simulink model "IEEE34bus_v2019b_Discrete_ZIPload"  (R2019b)
settings: Solver=ode4  StartTime=0.0  StopTime=5  FixedStep=Ts  MaxStep=1e-4  RelTol=1e-4
InitFcn:
  | a=1; % Loading Factor
  | Ts=50e-6;
  | % phase to sequence conversion of RXB matrices
  | c=1*exp(sqrt(-1)*(120*pi/180));
  | T=[1 1 1;1 c*c c;1 c c*c];
  | Tinv=1/3*[1 1 1;1 c c*c;1 c*c c];
  | 
  | % Simulation data for the IEEE 34 Node Test Feeder model
  | mi2km = 1.60934;%  miles to km conversion
  | ft2km = 0.0003048; % feet to km conversion
  | ms2F = 1*1e-6/(2*pi*60);% microsiemens to Farads conversion
  | 
  | %% Configuration 300 - series reactance - ohm/mile
  | R_300 = [1.3368 0.2101 0.2130;0.2101 1.3238 0.2066;0.2130 0.2066 1.3294];
  | X_300 = [1.3343 0.5779 0.5015;0.5779 1.3569 0.4591;0.5015 0.4591 1.3471];
  | % charging susceptance - microsiemens/mile
  | B_300 = [5.3350 -1.5313 -0.9943;-1.5313 5.0979 -0.6212;-0.9943 -0.6212 4.8880];
  | 
  | R_300 = R_300/mi2km;
  | Rseq=Tinv*R_300*T;
  | R1_300=Rseq(2,2);R0_300=Rseq(1,1);
  | 
  | L_300 = (X_300/(2*pi*60))/mi2km;
  | Lseq=Tinv*L_300*T;
  | L1_300=Lseq(2,2);L0_300=Lseq(1,1);
  | 
  | C_300 =(B_300*ms2F)/mi2km;
  | Cseq=Tinv*C_300*T;
  | C1_300=Cseq(2,2);C0_300=Cseq(1,1);
  | 
  | %% Configuration 301 - series reactance - ohm/mile
  | R_301 = [1.9300 0.2327 0.2359;0.2327 1.9157 0.2288;0.2359 0.2288 1.9219];
  | X_301 = [1.4115 0.6442 0.5691;0.6442 1.4281 0.5238;0.5691 0.5238 1.4209];
  | % charging susceptance - microsiemens/mile
  | B_301 = [5.1207 -1.4364 -0.9402;-1.4364 4.9055 -0.5951;-0.9402 -0.5951 4.7154];
  | 
  | R_301 = R_301/mi2km;
  | Rseq=Tinv*R_301*T;
  | R1_301=Rseq(2,2);R0_301=Rseq(1,1);
  | 
  | L_301 = (X_301/(2*pi*60))/mi2km;
  | Lseq=Tinv*L_301*T;
  | L1_301=Lseq(2,2);L0_301=Lseq(1,1);
  | 
  | C_301 =(B_301*ms2F)/mi2km;
  | Cseq=Tinv*C_301*T;
  | C1_301=Cseq(2,2);C0_301=Cseq(1,1);
  | 
  | %% Configuration 302 - series reactance - ohm/mile
  | R_302 = [2.7995 0 0;0 0 0;0 0 0];
  | X_302 = [1.4855 0 0;0 0 0;0 0 0];
  | % charging susceptance - microsiemens/mile
  | B_302 = [4.2251 0 0;0 0 0;0 0 0];
  | 
  | R_302 = R_302/mi2km;
  | Rseq=Tinv*R_302*T;
  | R1_302=Rseq(2,2);R0_302=Rseq(1,1);
  | 
  | L_302 = (X_302/(2*pi*60))/mi2km;
  | Lseq=Tinv*L_302*T;
  | ... (+41 lines)
undefined symbols (not defined in the file): find_system
libraries: powerlib x552, powerlib_meascontrol x162
(part 4 of 9)

== system IEEE34bus_v2019b_Discrete_ZIPload/836 D PQ ==
  "    1" : Gain  Gain=pi/180
  "    2" : Gain  Gain=pi/180
  "    3" : Gain  Gain=pi/180
  "    4" : Gain  Gain=1/sqrt(2)
  Clock : Clock
  Controlled Current Source : powerlib/Electrical Sources/Controlled Current Source  Initialize=off  Source_Type=AC  Amplitude=0  Phase=0  Frequency=0  Measurements=None
      settings: SourceProductName=Simscape Electrical
  Controlled Current Source1 : powerlib/Electrical Sources/Controlled Current Source  Initialize=off  Source_Type=AC  Amplitude=0  Phase=0  Frequency=0  Measurements=None
      settings: SourceProductName=Simscape Electrical
  Controlled Current Source2 : powerlib/Electrical Sources/Controlled Current Source  Initialize=off  Source_Type=AC  Amplitude=0  Phase=0  Frequency=0  Measurements=None
      settings: SourceProductName=Simscape Electrical
  Demux1 : Demux  Outputs=3
  Embedded MATLAB Function1 : MATLAB Function  TreatAsAtomicUnit=on
  Fourier : powerlib_meascontrol/Measurements/Fourier  Freq=fnom  n=1  InInit=[Vnom*sqrt(2) 0]  Ts=Ts
      settings: SourceProductName=Simscape Electrical
  Fourier1 : powerlib_meascontrol/Measurements/Fourier  Freq=60  n=1  InInit=[Vnom*sqrt(2) 0]  Ts=Ts
      settings: SourceProductName=Simscape Electrical
  Fourier2 : powerlib_meascontrol/Measurements/Fourier  Freq=60  n=1  InInit=[Vnom*sqrt(2) 0]  Ts=Ts
      settings: SourceProductName=Simscape Electrical
  Magnitude-Angle to Complex1 : MagnitudeAngleToComplex
  Memory3 : Memory
  Memory4 : Memory
  Mux : Mux  Inputs=3
  Rc+jXc1 : powerlib/Elements/Series RLC Branch  LConnTagsString=__new0  RConnTagsString=__new0  BranchType=R  Resistance=1e6  Inductance=1.6 / (120*pi) * 2  SetiL0=off  InitialCurrent=0  Capacitance=1e-6  Setx0=off  InitialVoltage=0  Measurements=None
      settings: SourceProductName=Simscape Electrical
  Rc+jXc2 : powerlib/Elements/Series RLC Branch  LConnTagsString=__new0  RConnTagsString=__new0  BranchType=R  Resistance=1e6  Inductance=1.6 / (120*pi) * 2  SetiL0=off  InitialCurrent=0  Capacitance=1e-6  Setx0=off  InitialVoltage=0  Measurements=None
      settings: SourceProductName=Simscape Electrical
  Rc+jXc3 : powerlib/Elements/Series RLC Branch  LConnTagsString=__new0  RConnTagsString=__new0  BranchType=R  Resistance=1e6  Inductance=1.6 / (120*pi) * 2  SetiL0=off  InitialCurrent=0  Capacitance=1e-6  Setx0=off  InitialVoltage=0  Measurements=None
      settings: SourceProductName=Simscape Electrical
  Sum : Sum  Inputs=|+-
  Voltage Measurement4 : powerlib/Measurements/Voltage Measurement  PhasorSimulation=off  OutputType=Complex  PSBequivalent=0
      settings: SourceProductName=Simscape Electrical
  Voltage Measurement5 : powerlib/Measurements/Voltage Measurement  PhasorSimulation=off  OutputType=Complex  PSBequivalent=0
      settings: SourceProductName=Simscape Electrical
  Voltage Measurement6 : powerlib/Measurements/Voltage Measurement  PhasorSimulation=off  OutputType=Complex  PSBequivalent=0
      settings: SourceProductName=Simscape Electrical
  " A" : PMIOPort  Tag=PMCPort  Side=Left
  " B" : PMIOPort  Tag=PMCPort  Port=2  Side=Left
  " C" : PMIOPort  Tag=PMCPort  Port=3  Side=Left
  wires:
  Magnitude-Angle to Complex1/1 -> Embedded MATLAB Function1/1(Vmeas)
  Memory3/1 -> Demux1/1, Fourier2/1
  "    4"/1 -> Magnitude-Angle to Complex1/1
  "    2"/1 -> Sum/1
  Voltage Measurement6/1 -> [vC]
  Demux1/1 -> Controlled Current Source/1
  [vC] -> Mux/3
  Sum/1 -> Memory4/1
  "    1"/1 -> Magnitude-Angle to Complex1/2
  Clock/1 -> Embedded MATLAB Function1/2(clock)
  Voltage Measurement5/1 -> [vB]
  Fourier1/2 -> "    2"/1
  Demux1/3 -> Controlled Current Source2/1
  Voltage Measurement4/1 -> [vA]
  Mux/1 -> Fourier/1
  Fourier/1 -> "    4"/1
  Demux1/2 -> Controlled Current Source1/1
  Fourier2/2 -> "    3"/1
  [del] -> Embedded MATLAB Function1/3(Ddel)
  Embedded MATLAB Function1/1(Iinjinst) -> Fourier1/1, Memory3/1
  [vA] -> Mux/1
  "    3"/1 -> Sum/2
  [vB] -> Mux/2
  Memory4/1 -> [del]
  Fourier/2 -> "    1"/1
  connections:
  Voltage Measurement5/LConn1 -- Rc+jXc2/LConn1 -- Controlled Current Source1/LConn1 -- " B"/RConn1 -- Rc+jXc1/RConn1 -- Controlled Current Source/RConn1 -- Voltage Measurement4/LConn2
  Voltage Measurement5/LConn2 -- Controlled Current Source1/RConn1 -- Rc+jXc2/RConn1 -- Controlled Current Source2/LConn1 -- " C"/RConn1 -- Voltage Measurement6/LConn1 -- Rc+jXc3/LConn1
  Voltage Measurement4/LConn1 -- Rc+jXc3/RConn1 -- Voltage Measurement6/LConn2 -- Controlled Current Source2/RConn1 -- Controlled Current Source/LConn1 -- " A"/RConn1 -- Rc+jXc1/LConn1

== system IEEE34bus_v2019b_Discrete_ZIPload/838 ==
  1 : powerlib/Measurements/Three-Phase V-I Measurement  VoltageMeasurement=phase-to-ground  SetLabelV=on  LabelV=V838  Vpu=off  VpuLL=off  CurrentMeasurement=no  SetLabelI=on  LabelI=I862  Ipu=off  Pbase=100e6  Vbase=24900  OutputType=Complex  PhasorSimulation=on  PSBequivalent=0
      settings: SourceProductName=Simscape Electrical
  Ground{1..2,9,12} (4 alike) : powerlib/Elements/Ground  LConnTagsString=a
      settings: SourceProductName=Simscape Electrical
  b : PMIOPort  Side=Left
  B : PMIOPort  Port=2  Side=Right
  connections:
  1/LConn2 -- B/RConn1
  Ground12/LConn1 -- 1/LConn1
  b/RConn1 -- 1/RConn2
  Ground9/LConn1 -- 1/RConn1
  Ground2/LConn1 -- 1/LConn3
  Ground1/LConn1 -- 1/RConn3

== system IEEE34bus_v2019b_Discrete_ZIPload/838 Y PQ ==
  "    1" : Gain  Gain=pi/180
  "    2" : Gain  Gain=pi/180
  "    3" : Gain  Gain=pi/180
  "    4" : Gain  Gain=1/sqrt(2)
  Clock : Clock
  Controlled Current Source : powerlib/Electrical Sources/Controlled Current Source  Initialize=off  Source_Type=AC  Amplitude=0  Phase=0  Frequency=0  Measurements=None
      settings: SourceProductName=Simscape Electrical
  Embedded MATLAB Function : MATLAB Function  TreatAsAtomicUnit=on
  Fourier : powerlib_meascontrol/Measurements/Fourier  Freq=60  n=1  InInit=[Vnom*sqrt(2) 0]  Ts=Ts
      settings: SourceProductName=Simscape Electrical
  Fourier1 : powerlib_meascontrol/Measurements/Fourier  Freq=60  n=1  InInit=[Vnom*sqrt(2) 0]  Ts=Ts
      settings: SourceProductName=Simscape Electrical
  Fourier2 : powerlib_meascontrol/Measurements/Fourier  Freq=60  n=1  InInit=[Vnom*sqrt(2) 0]  Ts=Ts
      settings: SourceProductName=Simscape Electrical
  Magnitude-Angle to Complex : MagnitudeAngleToComplex
  Memory1 : Memory
  Memory2 : Memory
  Rc+jXc1 : powerlib/Elements/Series RLC Branch  LConnTagsString=__new0  RConnTagsString=__new0  BranchType=R  Resistance=1e6  Inductance=1.6 / (120*pi) * 2  SetiL0=off  InitialCurrent=0  Capacitance=1e-6  Setx0=off  InitialVoltage=0  Measurements=None
      settings: SourceProductName=Simscape Electrical
  Sum : Sum  Inputs=|+-
  Voltage Measurement1 : powerlib/Measurements/Voltage Measurement  PhasorSimulation=off  OutputType=Complex  PSBequivalent=0
      settings: SourceProductName=Simscape Electrical
  " " : PMIOPort  Tag=PMCPort  Side=Left
  " 1" : PMIOPort  Tag=PMCPort  Port=2  Side=Right
  wires:
  Fourier1/2 -> "    1"/1
  Memory2/1 -> [del]
  Voltage Measurement1/1 -> [v]
  [v] -> Fourier/1
  "    1"/1 -> Sum/1
  Sum/1 -> Memory2/1
  Fourier/2 -> "    3"/1
  Fourier/1 -> "    4"/1
  [del] -> Embedded MATLAB Function/3(Ddel)
  Fourier2/2 -> "    2"/1
  Memory1/1 -> Controlled Current Source/1, Fourier2/1
  Embedded MATLAB Function/1(Iinjinst) -> Memory1/1, Fourier1/1
  Clock/1 -> Embedded MATLAB Function/2(clock)
  Magnitude-Angle to Complex/1 -> Embedded MATLAB Function/1(Vmeas)
  "    2"/1 -> Sum/2
  "    3"/1 -> Magnitude-Angle to Complex/2
  "    4"/1 -> Magnitude-Angle to Complex/1
  connections:
  " "/RConn1 -- Voltage Measurement1/LConn1 -- Controlled Current Source/LConn1 -- Rc+jXc1/LConn1
  Controlled Current Source/RConn1 -- Rc+jXc1/RConn1 -- Voltage Measurement1/LConn2 -- " 1"/RConn1

== system IEEE34bus_v2019b_Discrete_ZIPload/840 D I ==
  "    1" : Gain  Gain=pi/180
  "    2" : Gain  Gain=pi/180
  "    3" : Gain  Gain=pi/180
  "    4" : Gain  Gain=1/sqrt(2)
  Clock : Clock
  Controlled Current Source : powerlib/Electrical Sources/Controlled Current Source  Initialize=off  Source_Type=AC  Amplitude=0  Phase=0  Frequency=0  Measurements=None
      settings: SourceProductName=Simscape Electrical
  Controlled Current Source1 : powerlib/Electrical Sources/Controlled Current Source  Initialize=off  Source_Type=AC  Amplitude=0  Phase=0  Frequency=0  Measurements=None
      settings: SourceProductName=Simscape Electrical
  Controlled Current Source2 : powerlib/Electrical Sources/Controlled Current Source  Initialize=off  Source_Type=AC  Amplitude=0  Phase=0  Frequency=0  Measurements=None
      settings: SourceProductName=Simscape Electrical
  Demux1 : Demux  Outputs=3
  Embedded MATLAB Function1 : MATLAB Function  TreatAsAtomicUnit=on
  Fourier : powerlib_meascontrol/Measurements/Fourier  Freq=fnom  n=1  InInit=[Vnom*sqrt(2) 0]  Ts=Ts
      settings: SourceProductName=Simscape Electrical
  Fourier1 : powerlib_meascontrol/Measurements/Fourier  Freq=60  n=1  InInit=[Vnom*sqrt(2) 0]  Ts=Ts
      settings: SourceProductName=Simscape Electrical
  Fourier2 : powerlib_meascontrol/Measurements/Fourier  Freq=60  n=1  InInit=[Vnom*sqrt(2) 0]  Ts=Ts
      settings: SourceProductName=Simscape Electrical
  Magnitude-Angle to Complex1 : MagnitudeAngleToComplex
  Memory3 : Memory
  Memory4 : Memory
  Mux : Mux  Inputs=3
  Rc+jXc1 : powerlib/Elements/Series RLC Branch  LConnTagsString=__new0  RConnTagsString=__new0  BranchType=R  Resistance=1e6  Inductance=1.6 / (120*pi) * 2  SetiL0=off  InitialCurrent=0  Capacitance=1e-6  Setx0=off  InitialVoltage=0  Measurements=None
      settings: SourceProductName=Simscape Electrical
  Rc+jXc2 : powerlib/Elements/Series RLC Branch  LConnTagsString=__new0  RConnTagsString=__new0  BranchType=R  Resistance=1e6  Inductance=1.6 / (120*pi) * 2  SetiL0=off  InitialCurrent=0  Capacitance=1e-6  Setx0=off  InitialVoltage=0  Measurements=None
      settings: SourceProductName=Simscape Electrical
  Rc+jXc3 : powerlib/Elements/Series RLC Branch  LConnTagsString=__new0  RConnTagsString=__new0  BranchType=R  Resistance=1e6  Inductance=1.6 / (120*pi) * 2  SetiL0=off  InitialCurrent=0  Capacitance=1e-6  Setx0=off  InitialVoltage=0  Measurements=None
      settings: SourceProductName=Simscape Electrical
  Sum : Sum  Inputs=|+-
  Voltage Measurement4 : powerlib/Measurements/Voltage Measurement  PhasorSimulation=off  OutputType=Complex  PSBequivalent=0
      settings: SourceProductName=Simscape Electrical
  Voltage Measurement5 : powerlib/Measurements/Voltage Measurement  PhasorSimulation=off  OutputType=Complex  PSBequivalent=0
      settings: SourceProductName=Simscape Electrical
  Voltage Measurement6 : powerlib/Measurements/Voltage Measurement  PhasorSimulation=off  OutputType=Complex  PSBequivalent=0
      settings: SourceProductName=Simscape Electrical
  " A" : PMIOPort  Tag=PMCPort  Side=Left
  " B" : PMIOPort  Tag=PMCPort  Port=2  Side=Left
  " C" : PMIOPort  Tag=PMCPort  Port=3  Side=Left
  wires:
  Magnitude-Angle to Complex1/1 -> Embedded MATLAB Function1/1(Vmeas)
  Memory3/1 -> Demux1/1, Fourier2/1
  "    4"/1 -> Magnitude-Angle to Complex1/1
  "    2"/1 -> Sum/1
  Voltage Measurement6/1 -> [vC]
  Demux1/1 -> Controlled Current Source/1
  [vC] -> Mux/3
  Sum/1 -> Memory4/1
  "    1"/1 -> Magnitude-Angle to Complex1/2
  Clock/1 -> Embedded MATLAB Function1/2(clock)
  Voltage Measurement5/1 -> [vB]
  Fourier1/2 -> "    2"/1
  Demux1/3 -> Controlled Current Source2/1
  Voltage Measurement4/1 -> [vA]
  Mux/1 -> Fourier/1
  Fourier/1 -> "    4"/1
  Demux1/2 -> Controlled Current Source1/1
  Fourier2/2 -> "    3"/1
  [del] -> Embedded MATLAB Function1/3(Ddel)
  Embedded MATLAB Function1/1(Iinjinst) -> Fourier1/1, Memory3/1
  [vA] -> Mux/1
  "    3"/1 -> Sum/2
  [vB] -> Mux/2
  Memory4/1 -> [del]
  Fourier/2 -> "    1"/1
  connections:
  Voltage Measurement5/LConn1 -- Rc+jXc2/LConn1 -- Controlled Current Source1/LConn1 -- " B"/RConn1 -- Rc+jXc1/RConn1 -- Controlled Current Source/RConn1 -- Voltage Measurement4/LConn2
  Voltage Measurement5/LConn2 -- Controlled Current Source1/RConn1 -- Rc+jXc2/RConn1 -- Controlled Current Source2/LConn1 -- " C"/RConn1 -- Voltage Measurement6/LConn1 -- Rc+jXc3/LConn1
  Voltage Measurement4/LConn1 -- Rc+jXc3/RConn1 -- Voltage Measurement6/LConn2 -- Controlled Current Source2/RConn1 -- Controlled Current Source/LConn1 -- " A"/RConn1 -- Rc+jXc1/LConn1

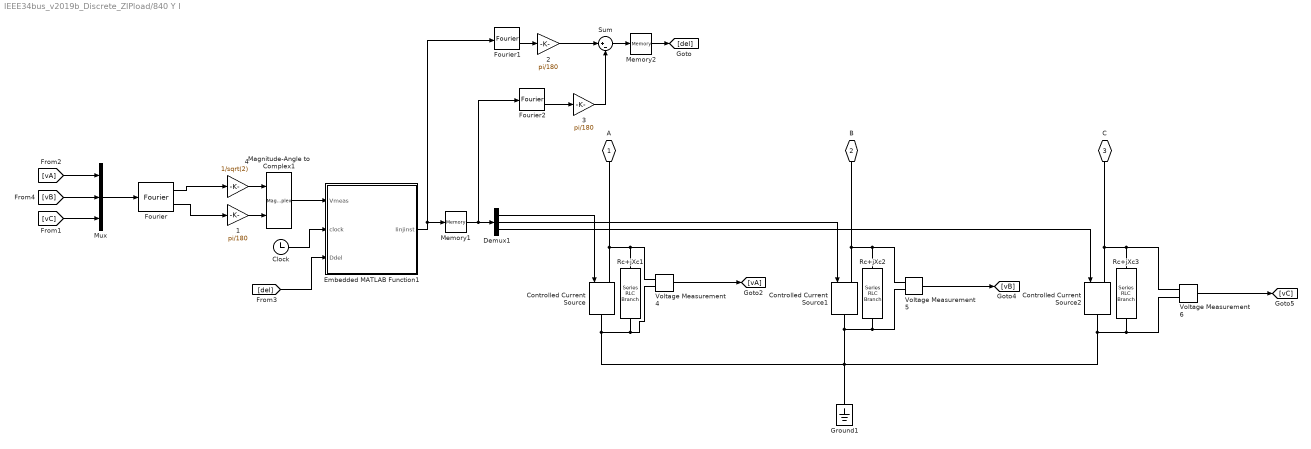
== system IEEE34bus_v2019b_Discrete_ZIPload/840 Y I ==
  "    1" : Gain  Gain=pi/180
  "    2" : Gain  Gain=pi/180
  "    3" : Gain  Gain=pi/180
  "    4" : Gain  Gain=1/sqrt(2)
  Clock : Clock
  Controlled Current Source : powerlib/Electrical Sources/Controlled Current Source  Initialize=off  Source_Type=AC  Amplitude=0  Phase=0  Frequency=0  Measurements=None
      settings: SourceProductName=Simscape Electrical
  Controlled Current Source1 : powerlib/Electrical Sources/Controlled Current Source  Initialize=off  Source_Type=AC  Amplitude=0  Phase=0  Frequency=0  Measurements=None
      settings: SourceProductName=Simscape Electrical
  Controlled Current Source2 : powerlib/Electrical Sources/Controlled Current Source  Initialize=off  Source_Type=AC  Amplitude=0  Phase=0  Frequency=0  Measurements=None
      settings: SourceProductName=Simscape Electrical
  Demux1 : Demux  Outputs=3
  Embedded MATLAB Function1 : MATLAB Function  TreatAsAtomicUnit=on
  Fourier : powerlib_meascontrol/Measurements/Fourier  Freq=fnom  n=1  InInit=[Vnom*sqrt(2) 0]  Ts=Ts
      settings: SourceProductName=Simscape Electrical
  Fourier1 : powerlib_meascontrol/Measurements/Fourier  Freq=60  n=1  InInit=[Vnom*sqrt(2) 0]  Ts=Ts
      settings: SourceProductName=Simscape Electrical
  Fourier2 : powerlib_meascontrol/Measurements/Fourier  Freq=60  n=1  InInit=[Vnom*sqrt(2) 0]  Ts=Ts
      settings: SourceProductName=Simscape Electrical
  Ground1 : powerlib/Elements/Ground  LConnTagsString=a
      settings: SourceProductName=Simscape Electrical
  Magnitude-Angle to Complex1 : MagnitudeAngleToComplex
  Memory1 : Memory
  Memory2 : Memory
  Mux : Mux  Inputs=3
  Rc+jXc1 : powerlib/Elements/Series RLC Branch  LConnTagsString=__new0  RConnTagsString=__new0  BranchType=R  Resistance=1e6  Inductance=1.6 / (120*pi) * 2  SetiL0=off  InitialCurrent=0  Capacitance=1e-6  Setx0=off  InitialVoltage=0  Measurements=None
      settings: SourceProductName=Simscape Electrical
  Rc+jXc2 : powerlib/Elements/Series RLC Branch  LConnTagsString=__new0  RConnTagsString=__new0  BranchType=R  Resistance=1e6  Inductance=1.6 / (120*pi) * 2  SetiL0=off  InitialCurrent=0  Capacitance=1e-6  Setx0=off  InitialVoltage=0  Measurements=None
      settings: SourceProductName=Simscape Electrical
  Rc+jXc3 : powerlib/Elements/Series RLC Branch  LConnTagsString=__new0  RConnTagsString=__new0  BranchType=R  Resistance=1e6  Inductance=1.6 / (120*pi) * 2  SetiL0=off  InitialCurrent=0  Capacitance=1e-6  Setx0=off  InitialVoltage=0  Measurements=None
      settings: SourceProductName=Simscape Electrical
  Sum : Sum  Inputs=|+-
  Voltage Measurement4 : powerlib/Measurements/Voltage Measurement  PhasorSimulation=off  OutputType=Complex  PSBequivalent=0
      settings: SourceProductName=Simscape Electrical
  Voltage Measurement5 : powerlib/Measurements/Voltage Measurement  PhasorSimulation=off  OutputType=Complex  PSBequivalent=0
      settings: SourceProductName=Simscape Electrical
  Voltage Measurement6 : powerlib/Measurements/Voltage Measurement  PhasorSimulation=off  OutputType=Complex  PSBequivalent=0
      settings: SourceProductName=Simscape Electrical
  " A" : PMIOPort  Tag=PMCPort  Side=Left
  " B" : PMIOPort  Tag=PMCPort  Port=2  Side=Left
  " C" : PMIOPort  Tag=PMCPort  Port=3  Side=Left
  wires:
  Voltage Measurement5/1 -> [vB]
  "    2"/1 -> Sum/1
  Magnitude-Angle to Complex1/1 -> Embedded MATLAB Function1/1(Vmeas)
  "    3"/1 -> Sum/2
  Memory1/1 -> Demux1/1, Fourier2/1
  Memory2/1 -> [del]
  Fourier/1 -> "    4"/1
  Fourier2/2 -> "    3"/1
  Voltage Measurement4/1 -> [vA]
  Voltage Measurement6/1 -> [vC]
  Demux1/2 -> Controlled Current Source1/1
  "    4"/1 -> Magnitude-Angle to Complex1/1
  Fourier1/2 -> "    2"/1
  Mux/1 -> Fourier/1
  Sum/1 -> Memory2/1
  [vA] -> Mux/1
  [vC] -> Mux/3
  [vB] -> Mux/2
  [del] -> Embedded MATLAB Function1/3(Ddel)
  Demux1/3 -> Controlled Current Source2/1
  Embedded MATLAB Function1/1(Iinjinst) -> Memory1/1, Fourier1/1
  Clock/1 -> Embedded MATLAB Function1/2(clock)
  Demux1/1 -> Controlled Current Source/1
  Fourier/2 -> "    1"/1
  "    1"/1 -> Magnitude-Angle to Complex1/2
  connections:
  Rc+jXc3/RConn1 -- Voltage Measurement6/LConn2 -- Voltage Measurement4/LConn2 -- Rc+jXc1/RConn1 -- Controlled Current Source/RConn1 -- Ground1/LConn1 -- Voltage Measurement5/LConn2 -- Rc+jXc2/RConn1 -- Controlled Current Source1/RConn1 -- Controlled Current Source2/RConn1
  Voltage Measurement4/LConn1 -- " A"/RConn1 -- Controlled Current Source/LConn1 -- Rc+jXc1/LConn1
  Voltage Measurement6/LConn1 -- Controlled Current Source2/LConn1 -- " C"/RConn1 -- Rc+jXc3/LConn1
  " B"/RConn1 -- Voltage Measurement5/LConn1 -- Rc+jXc2/LConn1 -- Controlled Current Source1/LConn1

== system IEEE34bus_v2019b_Discrete_ZIPload/842 Y PQ ==
  "    1" : Gain  Gain=pi/180
  "    2" : Gain  Gain=pi/180
  "    3" : Gain  Gain=pi/180
  "    4" : Gain  Gain=1/sqrt(2)
  Clock : Clock
  Controlled Current Source : powerlib/Electrical Sources/Controlled Current Source  Initialize=off  Source_Type=AC  Amplitude=0  Phase=0  Frequency=0  Measurements=None
      settings: SourceProductName=Simscape Electrical
  Embedded MATLAB Function : MATLAB Function  TreatAsAtomicUnit=on
  Fourier : powerlib_meascontrol/Measurements/Fourier  Freq=60  n=1  InInit=[Vnom*sqrt(2) 0]  Ts=Ts
      settings: SourceProductName=Simscape Electrical
  Fourier1 : powerlib_meascontrol/Measurements/Fourier  Freq=60  n=1  InInit=[Vnom*sqrt(2) 0]  Ts=Ts
      settings: SourceProductName=Simscape Electrical
  Fourier2 : powerlib_meascontrol/Measurements/Fourier  Freq=60  n=1  InInit=[Vnom*sqrt(2) 0]  Ts=Ts
      settings: SourceProductName=Simscape Electrical
  Magnitude-Angle to Complex : MagnitudeAngleToComplex
  Memory1 : Memory
  Memory2 : Memory
  Rc+jXc1 : powerlib/Elements/Series RLC Branch  LConnTagsString=__new0  RConnTagsString=__new0  BranchType=R  Resistance=1e6  Inductance=1.6 / (120*pi) * 2  SetiL0=off  InitialCurrent=0  Capacitance=1e-6  Setx0=off  InitialVoltage=0  Measurements=None
      settings: SourceProductName=Simscape Electrical
  Sum : Sum  Inputs=|+-
  Voltage Measurement1 : powerlib/Measurements/Voltage Measurement  PhasorSimulation=off  OutputType=Complex  PSBequivalent=0
      settings: SourceProductName=Simscape Electrical
  " " : PMIOPort  Tag=PMCPort  Side=Left
  " 1" : PMIOPort  Tag=PMCPort  Port=2  Side=Right
  wires:
  Fourier1/2 -> "    1"/1
  Memory2/1 -> [del]
  Voltage Measurement1/1 -> [v]
  [v] -> Fourier/1
  "    1"/1 -> Sum/1
  Sum/1 -> Memory2/1
  Fourier/2 -> "    3"/1
  Fourier/1 -> "    4"/1
  [del] -> Embedded MATLAB Function/3(Ddel)
  Fourier2/2 -> "    2"/1
  Memory1/1 -> Controlled Current Source/1, Fourier2/1
  Embedded MATLAB Function/1(Iinjinst) -> Memory1/1, Fourier1/1
  Clock/1 -> Embedded MATLAB Function/2(clock)
  Magnitude-Angle to Complex/1 -> Embedded MATLAB Function/1(Vmeas)
  "    2"/1 -> Sum/2
  "    3"/1 -> Magnitude-Angle to Complex/2
  "    4"/1 -> Magnitude-Angle to Complex/1
  connections:
  " "/RConn1 -- Voltage Measurement1/LConn1 -- Controlled Current Source/LConn1 -- Rc+jXc1/LConn1
  Controlled Current Source/RConn1 -- Rc+jXc1/RConn1 -- Voltage Measurement1/LConn2 -- " 1"/RConn1

== system IEEE34bus_v2019b_Discrete_ZIPload/844 Y PQ ==
  "    1" : Gain  Gain=pi/180
  "    2" : Gain  Gain=pi/180
  "    3" : Gain  Gain=pi/180
  "    4" : Gain  Gain=1/sqrt(2)
  Clock : Clock
  Controlled Current Source : powerlib/Electrical Sources/Controlled Current Source  Initialize=off  Source_Type=AC  Amplitude=0  Phase=0  Frequency=0  Measurements=None
      settings: SourceProductName=Simscape Electrical
  Embedded MATLAB Function : MATLAB Function  TreatAsAtomicUnit=on
  Fourier : powerlib_meascontrol/Measurements/Fourier  Freq=60  n=1  InInit=[Vnom*sqrt(2) 0]  Ts=Ts
      settings: SourceProductName=Simscape Electrical
  Fourier1 : powerlib_meascontrol/Measurements/Fourier  Freq=60  n=1  InInit=[Vnom*sqrt(2) 0]  Ts=Ts
      settings: SourceProductName=Simscape Electrical
  Fourier2 : powerlib_meascontrol/Measurements/Fourier  Freq=60  n=1  InInit=[Vnom*sqrt(2) 0]  Ts=Ts
      settings: SourceProductName=Simscape Electrical
  Magnitude-Angle to Complex : MagnitudeAngleToComplex
  Memory1 : Memory
  Memory2 : Memory
  Rc+jXc1 : powerlib/Elements/Series RLC Branch  LConnTagsString=__new0  RConnTagsString=__new0  BranchType=R  Resistance=1e6  Inductance=1.6 / (120*pi) * 2  SetiL0=off  InitialCurrent=0  Capacitance=1e-6  Setx0=off  InitialVoltage=0  Measurements=None
      settings: SourceProductName=Simscape Electrical
  Sum : Sum  Inputs=|+-
  Voltage Measurement1 : powerlib/Measurements/Voltage Measurement  PhasorSimulation=off  OutputType=Complex  PSBequivalent=0
      settings: SourceProductName=Simscape Electrical
  " " : PMIOPort  Tag=PMCPort  Side=Left
  " 1" : PMIOPort  Tag=PMCPort  Port=2  Side=Right
  wires:
  Fourier1/2 -> "    1"/1
  Memory2/1 -> [del]
  Voltage Measurement1/1 -> [v]
  [v] -> Fourier/1
  "    1"/1 -> Sum/1
  Sum/1 -> Memory2/1
  Fourier/2 -> "    3"/1
  Fourier/1 -> "    4"/1
  [del] -> Embedded MATLAB Function/3(Ddel)
  Fourier2/2 -> "    2"/1
  Memory1/1 -> Controlled Current Source/1, Fourier2/1
  Embedded MATLAB Function/1(Iinjinst) -> Memory1/1, Fourier1/1
  Clock/1 -> Embedded MATLAB Function/2(clock)
  Magnitude-Angle to Complex/1 -> Embedded MATLAB Function/1(Vmeas)
  "    2"/1 -> Sum/2
  "    3"/1 -> Magnitude-Angle to Complex/2
  "    4"/1 -> Magnitude-Angle to Complex/1
  connections:
  " "/RConn1 -- Voltage Measurement1/LConn1 -- Controlled Current Source/LConn1 -- Rc+jXc1/LConn1
  Controlled Current Source/RConn1 -- Rc+jXc1/RConn1 -- Voltage Measurement1/LConn2 -- " 1"/RConn1

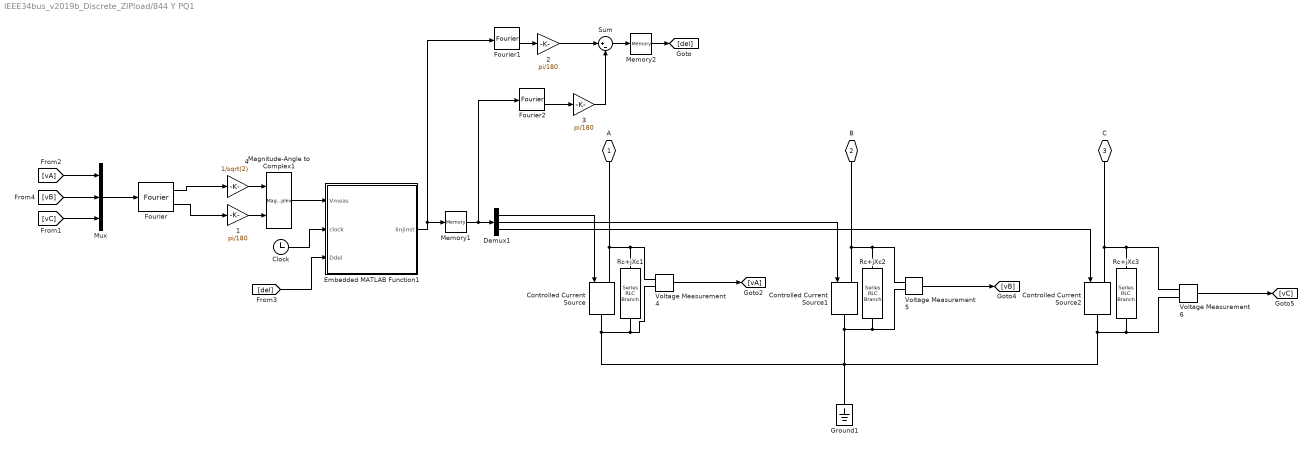
== system IEEE34bus_v2019b_Discrete_ZIPload/844 Y PQ1 ==
  "    1" : Gain  Gain=pi/180
  "    2" : Gain  Gain=pi/180
  "    3" : Gain  Gain=pi/180
  "    4" : Gain  Gain=1/sqrt(2)
  Clock : Clock
  Controlled Current Source : powerlib/Electrical Sources/Controlled Current Source  Initialize=off  Source_Type=AC  Amplitude=0  Phase=0  Frequency=0  Measurements=None
      settings: SourceProductName=Simscape Electrical
  Controlled Current Source1 : powerlib/Electrical Sources/Controlled Current Source  Initialize=off  Source_Type=AC  Amplitude=0  Phase=0  Frequency=0  Measurements=None
      settings: SourceProductName=Simscape Electrical
  Controlled Current Source2 : powerlib/Electrical Sources/Controlled Current Source  Initialize=off  Source_Type=AC  Amplitude=0  Phase=0  Frequency=0  Measurements=None
      settings: SourceProductName=Simscape Electrical
  Demux1 : Demux  Outputs=3
  Embedded MATLAB Function1 : MATLAB Function  TreatAsAtomicUnit=on
  Fourier : powerlib_meascontrol/Measurements/Fourier  Freq=fnom  n=1  InInit=[Vnom*sqrt(2) 0]  Ts=Ts
      settings: SourceProductName=Simscape Electrical
  Fourier1 : powerlib_meascontrol/Measurements/Fourier  Freq=60  n=1  InInit=[Vnom*sqrt(2) 0]  Ts=Ts
      settings: SourceProductName=Simscape Electrical
  Fourier2 : powerlib_meascontrol/Measurements/Fourier  Freq=60  n=1  InInit=[Vnom*sqrt(2) 0]  Ts=Ts
      settings: SourceProductName=Simscape Electrical
  Ground1 : powerlib/Elements/Ground  LConnTagsString=a
      settings: SourceProductName=Simscape Electrical
  Magnitude-Angle to Complex1 : MagnitudeAngleToComplex
  Memory1 : Memory
  Memory2 : Memory
  Mux : Mux  Inputs=3
  Rc+jXc1 : powerlib/Elements/Series RLC Branch  LConnTagsString=__new0  RConnTagsString=__new0  BranchType=R  Resistance=1e6  Inductance=1.6 / (120*pi) * 2  SetiL0=off  InitialCurrent=0  Capacitance=1e-6  Setx0=off  InitialVoltage=0  Measurements=None
      settings: SourceProductName=Simscape Electrical
  Rc+jXc2 : powerlib/Elements/Series RLC Branch  LConnTagsString=__new0  RConnTagsString=__new0  BranchType=R  Resistance=1e6  Inductance=1.6 / (120*pi) * 2  SetiL0=off  InitialCurrent=0  Capacitance=1e-6  Setx0=off  InitialVoltage=0  Measurements=None
      settings: SourceProductName=Simscape Electrical
  Rc+jXc3 : powerlib/Elements/Series RLC Branch  LConnTagsString=__new0  RConnTagsString=__new0  BranchType=R  Resistance=1e6  Inductance=1.6 / (120*pi) * 2  SetiL0=off  InitialCurrent=0  Capacitance=1e-6  Setx0=off  InitialVoltage=0  Measurements=None
      settings: SourceProductName=Simscape Electrical
  Sum : Sum  Inputs=|+-
  Voltage Measurement4 : powerlib/Measurements/Voltage Measurement  PhasorSimulation=off  OutputType=Complex  PSBequivalent=0
      settings: SourceProductName=Simscape Electrical
  Voltage Measurement5 : powerlib/Measurements/Voltage Measurement  PhasorSimulation=off  OutputType=Complex  PSBequivalent=0
      settings: SourceProductName=Simscape Electrical
  Voltage Measurement6 : powerlib/Measurements/Voltage Measurement  PhasorSimulation=off  OutputType=Complex  PSBequivalent=0
      settings: SourceProductName=Simscape Electrical
  " A" : PMIOPort  Tag=PMCPort  Side=Left
  " B" : PMIOPort  Tag=PMCPort  Port=2  Side=Left
  " C" : PMIOPort  Tag=PMCPort  Port=3  Side=Left
  wires:
  Voltage Measurement5/1 -> [vB]
  "    2"/1 -> Sum/1
  Magnitude-Angle to Complex1/1 -> Embedded MATLAB Function1/1(Vmeas)
  "    3"/1 -> Sum/2
  Memory1/1 -> Demux1/1, Fourier2/1
  Memory2/1 -> [del]
  Fourier/1 -> "    4"/1
  Fourier2/2 -> "    3"/1
  Voltage Measurement4/1 -> [vA]
  Voltage Measurement6/1 -> [vC]
  Demux1/2 -> Controlled Current Source1/1
  "    4"/1 -> Magnitude-Angle to Complex1/1
  Fourier1/2 -> "    2"/1
  Mux/1 -> Fourier/1
  Sum/1 -> Memory2/1
  [vA] -> Mux/1
  [vC] -> Mux/3
  [vB] -> Mux/2
  [del] -> Embedded MATLAB Function1/3(Ddel)
  Demux1/3 -> Controlled Current Source2/1
  Embedded MATLAB Function1/1(Iinjinst) -> Memory1/1, Fourier1/1
  Clock/1 -> Embedded MATLAB Function1/2(clock)
  Demux1/1 -> Controlled Current Source/1
  Fourier/2 -> "    1"/1
  "    1"/1 -> Magnitude-Angle to Complex1/2
  connections:
  Rc+jXc3/RConn1 -- Voltage Measurement6/LConn2 -- Voltage Measurement4/LConn2 -- Rc+jXc1/RConn1 -- Controlled Current Source/RConn1 -- Ground1/LConn1 -- Voltage Measurement5/LConn2 -- Rc+jXc2/RConn1 -- Controlled Current Source1/RConn1 -- Controlled Current Source2/RConn1
  Voltage Measurement4/LConn1 -- " A"/RConn1 -- Controlled Current Source/LConn1 -- Rc+jXc1/LConn1
  Voltage Measurement6/LConn1 -- Controlled Current Source2/LConn1 -- " C"/RConn1 -- Rc+jXc3/LConn1
  " B"/RConn1 -- Voltage Measurement5/LConn1 -- Rc+jXc2/LConn1 -- Controlled Current Source1/LConn1

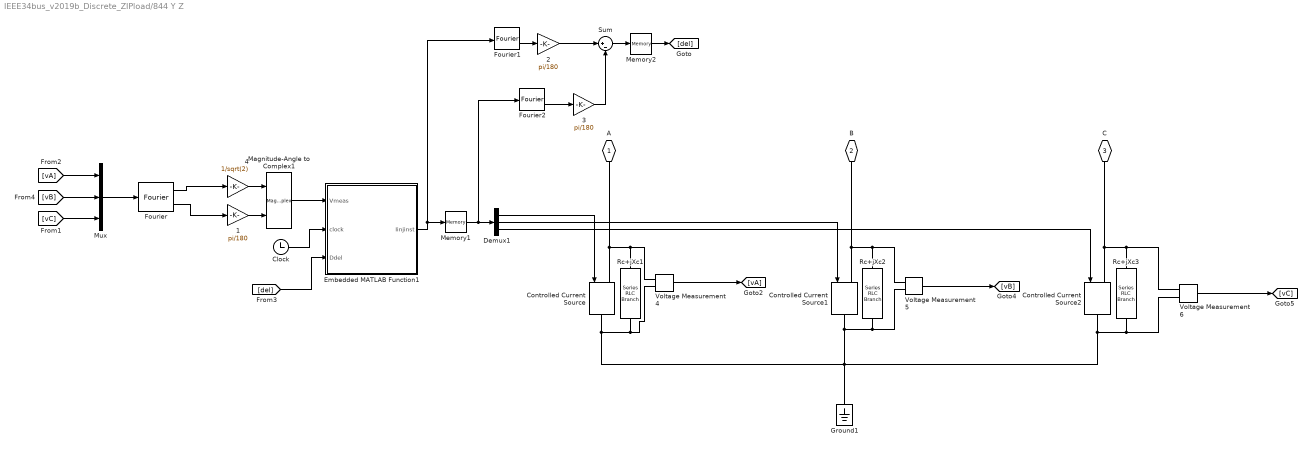
== system IEEE34bus_v2019b_Discrete_ZIPload/844 Y Z ==
  "    1" : Gain  Gain=pi/180
  "    2" : Gain  Gain=pi/180
  "    3" : Gain  Gain=pi/180
  "    4" : Gain  Gain=1/sqrt(2)
  Clock : Clock
  Controlled Current Source : powerlib/Electrical Sources/Controlled Current Source  Initialize=off  Source_Type=AC  Amplitude=0  Phase=0  Frequency=0  Measurements=None
      settings: SourceProductName=Simscape Electrical
  Controlled Current Source1 : powerlib/Electrical Sources/Controlled Current Source  Initialize=off  Source_Type=AC  Amplitude=0  Phase=0  Frequency=0  Measurements=None
      settings: SourceProductName=Simscape Electrical
  Controlled Current Source2 : powerlib/Electrical Sources/Controlled Current Source  Initialize=off  Source_Type=AC  Amplitude=0  Phase=0  Frequency=0  Measurements=None
      settings: SourceProductName=Simscape Electrical
  Demux1 : Demux  Outputs=3
  Embedded MATLAB Function1 : MATLAB Function  TreatAsAtomicUnit=on
  Fourier : powerlib_meascontrol/Measurements/Fourier  Freq=fnom  n=1  InInit=[Vnom*sqrt(2) 0]  Ts=Ts
      settings: SourceProductName=Simscape Electrical
  Fourier1 : powerlib_meascontrol/Measurements/Fourier  Freq=60  n=1  InInit=[Vnom*sqrt(2) 0]  Ts=Ts
      settings: SourceProductName=Simscape Electrical
  Fourier2 : powerlib_meascontrol/Measurements/Fourier  Freq=60  n=1  InInit=[Vnom*sqrt(2) 0]  Ts=Ts
      settings: SourceProductName=Simscape Electrical
  Ground1 : powerlib/Elements/Ground  LConnTagsString=a
      settings: SourceProductName=Simscape Electrical
  Magnitude-Angle to Complex1 : MagnitudeAngleToComplex
  Memory1 : Memory
  Memory2 : Memory
  Mux : Mux  Inputs=3
  Rc+jXc1 : powerlib/Elements/Series RLC Branch  LConnTagsString=__new0  RConnTagsString=__new0  BranchType=R  Resistance=1e6  Inductance=1.6 / (120*pi) * 2  SetiL0=off  InitialCurrent=0  Capacitance=1e-6  Setx0=off  InitialVoltage=0  Measurements=None
      settings: SourceProductName=Simscape Electrical
  Rc+jXc2 : powerlib/Elements/Series RLC Branch  LConnTagsString=__new0  RConnTagsString=__new0  BranchType=R  Resistance=1e6  Inductance=1.6 / (120*pi) * 2  SetiL0=off  InitialCurrent=0  Capacitance=1e-6  Setx0=off  InitialVoltage=0  Measurements=None
      settings: SourceProductName=Simscape Electrical
  Rc+jXc3 : powerlib/Elements/Series RLC Branch  LConnTagsString=__new0  RConnTagsString=__new0  BranchType=R  Resistance=1e6  Inductance=1.6 / (120*pi) * 2  SetiL0=off  InitialCurrent=0  Capacitance=1e-6  Setx0=off  InitialVoltage=0  Measurements=None
      settings: SourceProductName=Simscape Electrical
  Sum : Sum  Inputs=|+-
  Voltage Measurement4 : powerlib/Measurements/Voltage Measurement  PhasorSimulation=off  OutputType=Complex  PSBequivalent=0
      settings: SourceProductName=Simscape Electrical
  Voltage Measurement5 : powerlib/Measurements/Voltage Measurement  PhasorSimulation=off  OutputType=Complex  PSBequivalent=0
      settings: SourceProductName=Simscape Electrical
  Voltage Measurement6 : powerlib/Measurements/Voltage Measurement  PhasorSimulation=off  OutputType=Complex  PSBequivalent=0
      settings: SourceProductName=Simscape Electrical
  " A" : PMIOPort  Tag=PMCPort  Side=Left
  " B" : PMIOPort  Tag=PMCPort  Port=2  Side=Left
  " C" : PMIOPort  Tag=PMCPort  Port=3  Side=Left
  wires:
  Voltage Measurement5/1 -> [vB]
  "    2"/1 -> Sum/1
  Magnitude-Angle to Complex1/1 -> Embedded MATLAB Function1/1(Vmeas)
  "    3"/1 -> Sum/2
  Memory1/1 -> Demux1/1, Fourier2/1
  Memory2/1 -> [del]
  Fourier/1 -> "    4"/1
  Fourier2/2 -> "    3"/1
  Voltage Measurement4/1 -> [vA]
  Voltage Measurement6/1 -> [vC]
  Demux1/2 -> Controlled Current Source1/1
  "    4"/1 -> Magnitude-Angle to Complex1/1
  Fourier1/2 -> "    2"/1
  Mux/1 -> Fourier/1
  Sum/1 -> Memory2/1
  [vA] -> Mux/1
  [vC] -> Mux/3
  [vB] -> Mux/2
  [del] -> Embedded MATLAB Function1/3(Ddel)
  Demux1/3 -> Controlled Current Source2/1
  Embedded MATLAB Function1/1(Iinjinst) -> Memory1/1, Fourier1/1
  Clock/1 -> Embedded MATLAB Function1/2(clock)
  Demux1/1 -> Controlled Current Source/1
  Fourier/2 -> "    1"/1
  "    1"/1 -> Magnitude-Angle to Complex1/2
  connections:
  Rc+jXc3/RConn1 -- Voltage Measurement6/LConn2 -- Voltage Measurement4/LConn2 -- Rc+jXc1/RConn1 -- Controlled Current Source/RConn1 -- Ground1/LConn1 -- Voltage Measurement5/LConn2 -- Rc+jXc2/RConn1 -- Controlled Current Source1/RConn1 -- Controlled Current Source2/RConn1
  Voltage Measurement4/LConn1 -- " A"/RConn1 -- Controlled Current Source/LConn1 -- Rc+jXc1/LConn1
  Voltage Measurement6/LConn1 -- Controlled Current Source2/LConn1 -- " C"/RConn1 -- Rc+jXc3/LConn1
  " B"/RConn1 -- Voltage Measurement5/LConn1 -- Rc+jXc2/LConn1 -- Controlled Current Source1/LConn1

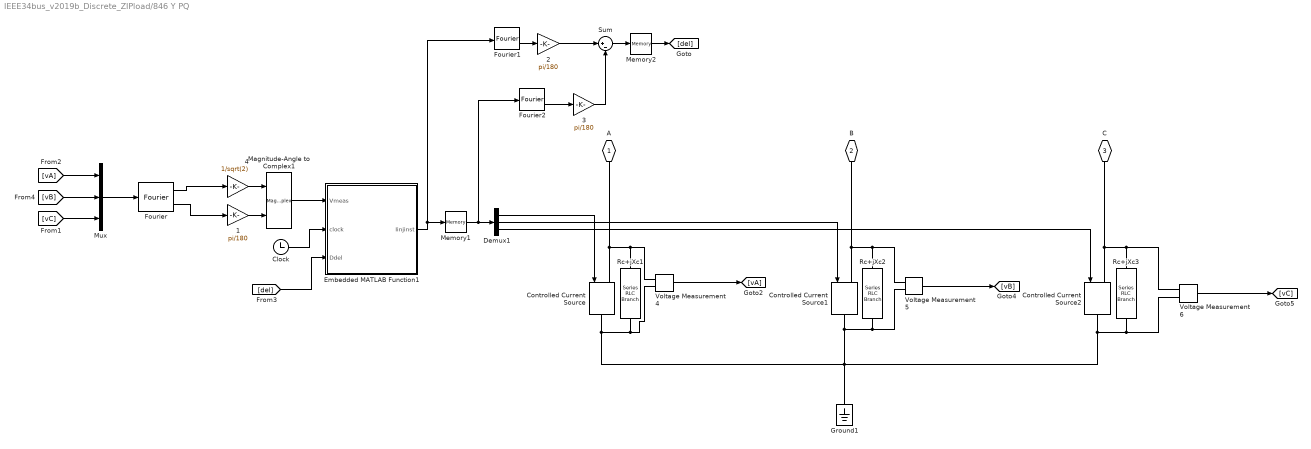
== system IEEE34bus_v2019b_Discrete_ZIPload/846 Y PQ ==
  "    1" : Gain  Gain=pi/180
  "    2" : Gain  Gain=pi/180
  "    3" : Gain  Gain=pi/180
  "    4" : Gain  Gain=1/sqrt(2)
  Clock : Clock
  Controlled Current Source : powerlib/Electrical Sources/Controlled Current Source  Initialize=off  Source_Type=AC  Amplitude=0  Phase=0  Frequency=0  Measurements=None
      settings: SourceProductName=Simscape Electrical
  Controlled Current Source1 : powerlib/Electrical Sources/Controlled Current Source  Initialize=off  Source_Type=AC  Amplitude=0  Phase=0  Frequency=0  Measurements=None
      settings: SourceProductName=Simscape Electrical
  Controlled Current Source2 : powerlib/Electrical Sources/Controlled Current Source  Initialize=off  Source_Type=AC  Amplitude=0  Phase=0  Frequency=0  Measurements=None
      settings: SourceProductName=Simscape Electrical
  Demux1 : Demux  Outputs=3
  Embedded MATLAB Function1 : MATLAB Function  TreatAsAtomicUnit=on
  Fourier : powerlib_meascontrol/Measurements/Fourier  Freq=fnom  n=1  InInit=[Vnom*sqrt(2) 0]  Ts=Ts
      settings: SourceProductName=Simscape Electrical
  Fourier1 : powerlib_meascontrol/Measurements/Fourier  Freq=60  n=1  InInit=[Vnom*sqrt(2) 0]  Ts=Ts
      settings: SourceProductName=Simscape Electrical
  Fourier2 : powerlib_meascontrol/Measurements/Fourier  Freq=60  n=1  InInit=[Vnom*sqrt(2) 0]  Ts=Ts
      settings: SourceProductName=Simscape Electrical
  Ground1 : powerlib/Elements/Ground  LConnTagsString=a
      settings: SourceProductName=Simscape Electrical
  Magnitude-Angle to Complex1 : MagnitudeAngleToComplex
  Memory1 : Memory
  Memory2 : Memory
  Mux : Mux  Inputs=3
  Rc+jXc1 : powerlib/Elements/Series RLC Branch  LConnTagsString=__new0  RConnTagsString=__new0  BranchType=R  Resistance=1e6  Inductance=1.6 / (120*pi) * 2  SetiL0=off  InitialCurrent=0  Capacitance=1e-6  Setx0=off  InitialVoltage=0  Measurements=None
      settings: SourceProductName=Simscape Electrical
  Rc+jXc2 : powerlib/Elements/Series RLC Branch  LConnTagsString=__new0  RConnTagsString=__new0  BranchType=R  Resistance=1e6  Inductance=1.6 / (120*pi) * 2  SetiL0=off  InitialCurrent=0  Capacitance=1e-6  Setx0=off  InitialVoltage=0  Measurements=None
      settings: SourceProductName=Simscape Electrical
  Rc+jXc3 : powerlib/Elements/Series RLC Branch  LConnTagsString=__new0  RConnTagsString=__new0  BranchType=R  Resistance=1e6  Inductance=1.6 / (120*pi) * 2  SetiL0=off  InitialCurrent=0  Capacitance=1e-6  Setx0=off  InitialVoltage=0  Measurements=None
      settings: SourceProductName=Simscape Electrical
  Sum : Sum  Inputs=|+-
  Voltage Measurement4 : powerlib/Measurements/Voltage Measurement  PhasorSimulation=off  OutputType=Complex  PSBequivalent=0
      settings: SourceProductName=Simscape Electrical
  Voltage Measurement5 : powerlib/Measurements/Voltage Measurement  PhasorSimulation=off  OutputType=Complex  PSBequivalent=0
      settings: SourceProductName=Simscape Electrical
  Voltage Measurement6 : powerlib/Measurements/Voltage Measurement  PhasorSimulation=off  OutputType=Complex  PSBequivalent=0
      settings: SourceProductName=Simscape Electrical
  " A" : PMIOPort  Tag=PMCPort  Side=Left
  " B" : PMIOPort  Tag=PMCPort  Port=2  Side=Left
  " C" : PMIOPort  Tag=PMCPort  Port=3  Side=Left
  wires:
  Voltage Measurement5/1 -> [vB]
  "    2"/1 -> Sum/1
  Magnitude-Angle to Complex1/1 -> Embedded MATLAB Function1/1(Vmeas)
  "    3"/1 -> Sum/2
  Memory1/1 -> Demux1/1, Fourier2/1
  Memory2/1 -> [del]
  Fourier/1 -> "    4"/1
  Fourier2/2 -> "    3"/1
  Voltage Measurement4/1 -> [vA]
  Voltage Measurement6/1 -> [vC]
  Demux1/2 -> Controlled Current Source1/1
  "    4"/1 -> Magnitude-Angle to Complex1/1
  Fourier1/2 -> "    2"/1
  Mux/1 -> Fourier/1
  Sum/1 -> Memory2/1
  [vA] -> Mux/1
  [vC] -> Mux/3
  [vB] -> Mux/2
  [del] -> Embedded MATLAB Function1/3(Ddel)
  Demux1/3 -> Controlled Current Source2/1
  Embedded MATLAB Function1/1(Iinjinst) -> Memory1/1, Fourier1/1
  Clock/1 -> Embedded MATLAB Function1/2(clock)
  Demux1/1 -> Controlled Current Source/1
  Fourier/2 -> "    1"/1
  "    1"/1 -> Magnitude-Angle to Complex1/2
  connections:
  Rc+jXc3/RConn1 -- Voltage Measurement6/LConn2 -- Voltage Measurement4/LConn2 -- Rc+jXc1/RConn1 -- Controlled Current Source/RConn1 -- Ground1/LConn1 -- Voltage Measurement5/LConn2 -- Rc+jXc2/RConn1 -- Controlled Current Source1/RConn1 -- Controlled Current Source2/RConn1
  Voltage Measurement4/LConn1 -- " A"/RConn1 -- Controlled Current Source/LConn1 -- Rc+jXc1/LConn1
  Voltage Measurement6/LConn1 -- Controlled Current Source2/LConn1 -- " C"/RConn1 -- Rc+jXc3/LConn1
  " B"/RConn1 -- Voltage Measurement5/LConn1 -- Rc+jXc2/LConn1 -- Controlled Current Source1/LConn1

== system IEEE34bus_v2019b_Discrete_ZIPload/846 Y PQ1 ==
  "    1" : Gain  Gain=pi/180
  "    2" : Gain  Gain=pi/180
  "    3" : Gain  Gain=pi/180
  "    4" : Gain  Gain=1/sqrt(2)
  Clock : Clock
  Controlled Current Source : powerlib/Electrical Sources/Controlled Current Source  Initialize=off  Source_Type=AC  Amplitude=0  Phase=0  Frequency=0  Measurements=None
      settings: SourceProductName=Simscape Electrical
  Embedded MATLAB Function : MATLAB Function  TreatAsAtomicUnit=on
  Fourier : powerlib_meascontrol/Measurements/Fourier  Freq=60  n=1  InInit=[Vnom*sqrt(2) 0]  Ts=Ts
      settings: SourceProductName=Simscape Electrical
  Fourier1 : powerlib_meascontrol/Measurements/Fourier  Freq=60  n=1  InInit=[Vnom*sqrt(2) 0]  Ts=Ts
      settings: SourceProductName=Simscape Electrical
  Fourier2 : powerlib_meascontrol/Measurements/Fourier  Freq=60  n=1  InInit=[Vnom*sqrt(2) 0]  Ts=Ts
      settings: SourceProductName=Simscape Electrical
  Magnitude-Angle to Complex : MagnitudeAngleToComplex
  Memory1 : Memory
  Memory2 : Memory
  Rc+jXc1 : powerlib/Elements/Series RLC Branch  LConnTagsString=__new0  RConnTagsString=__new0  BranchType=R  Resistance=1e6  Inductance=1.6 / (120*pi) * 2  SetiL0=off  InitialCurrent=0  Capacitance=1e-6  Setx0=off  InitialVoltage=0  Measurements=None
      settings: SourceProductName=Simscape Electrical
  Sum : Sum  Inputs=|+-
  Voltage Measurement1 : powerlib/Measurements/Voltage Measurement  PhasorSimulation=off  OutputType=Complex  PSBequivalent=0
      settings: SourceProductName=Simscape Electrical
  " " : PMIOPort  Tag=PMCPort  Side=Left
  " 1" : PMIOPort  Tag=PMCPort  Port=2  Side=Right
  wires:
  Fourier1/2 -> "    1"/1
  Memory2/1 -> [del]
  Voltage Measurement1/1 -> [v]
  [v] -> Fourier/1
  "    1"/1 -> Sum/1
  Sum/1 -> Memory2/1
  Fourier/2 -> "    3"/1
  Fourier/1 -> "    4"/1
  [del] -> Embedded MATLAB Function/3(Ddel)
  Fourier2/2 -> "    2"/1
  Memory1/1 -> Controlled Current Source/1, Fourier2/1
  Embedded MATLAB Function/1(Iinjinst) -> Memory1/1, Fourier1/1
  Clock/1 -> Embedded MATLAB Function/2(clock)
  Magnitude-Angle to Complex/1 -> Embedded MATLAB Function/1(Vmeas)
  "    2"/1 -> Sum/2
  "    3"/1 -> Magnitude-Angle to Complex/2
  "    4"/1 -> Magnitude-Angle to Complex/1
  connections:
  " "/RConn1 -- Voltage Measurement1/LConn1 -- Controlled Current Source/LConn1 -- Rc+jXc1/LConn1
  Controlled Current Source/RConn1 -- Rc+jXc1/RConn1 -- Voltage Measurement1/LConn2 -- " 1"/RConn1

== system IEEE34bus_v2019b_Discrete_ZIPload/848 D PQ ==
  "    1" : Gain  Gain=pi/180
  "    2" : Gain  Gain=pi/180
  "    3" : Gain  Gain=pi/180
  "    4" : Gain  Gain=1/sqrt(2)
  Clock : Clock
  Controlled Current Source : powerlib/Electrical Sources/Controlled Current Source  Initialize=off  Source_Type=AC  Amplitude=0  Phase=0  Frequency=0  Measurements=None
      settings: SourceProductName=Simscape Electrical
  Controlled Current Source1 : powerlib/Electrical Sources/Controlled Current Source  Initialize=off  Source_Type=AC  Amplitude=0  Phase=0  Frequency=0  Measurements=None
      settings: SourceProductName=Simscape Electrical
  Controlled Current Source2 : powerlib/Electrical Sources/Controlled Current Source  Initialize=off  Source_Type=AC  Amplitude=0  Phase=0  Frequency=0  Measurements=None
      settings: SourceProductName=Simscape Electrical
  Demux1 : Demux  Outputs=3
  Embedded MATLAB Function1 : MATLAB Function  TreatAsAtomicUnit=on
  Fourier : powerlib_meascontrol/Measurements/Fourier  Freq=fnom  n=1  InInit=[Vnom*sqrt(2) 0]  Ts=Ts
      settings: SourceProductName=Simscape Electrical
  Fourier1 : powerlib_meascontrol/Measurements/Fourier  Freq=60  n=1  InInit=[Vnom*sqrt(2) 0]  Ts=Ts
      settings: SourceProductName=Simscape Electrical
  Fourier2 : powerlib_meascontrol/Measurements/Fourier  Freq=60  n=1  InInit=[Vnom*sqrt(2) 0]  Ts=Ts
      settings: SourceProductName=Simscape Electrical
  Magnitude-Angle to Complex1 : MagnitudeAngleToComplex
  Memory3 : Memory
  Memory4 : Memory
  Mux : Mux  Inputs=3
  Rc+jXc1 : powerlib/Elements/Series RLC Branch  LConnTagsString=__new0  RConnTagsString=__new0  BranchType=R  Resistance=1e6  Inductance=1.6 / (120*pi) * 2  SetiL0=off  InitialCurrent=0  Capacitance=1e-6  Setx0=off  InitialVoltage=0  Measurements=None
      settings: SourceProductName=Simscape Electrical
  Rc+jXc2 : powerlib/Elements/Series RLC Branch  LConnTagsString=__new0  RConnTagsString=__new0  BranchType=R  Resistance=1e6  Inductance=1.6 / (120*pi) * 2  SetiL0=off  InitialCurrent=0  Capacitance=1e-6  Setx0=off  InitialVoltage=0  Measurements=None
      settings: SourceProductName=Simscape Electrical
  Rc+jXc3 : powerlib/Elements/Series RLC Branch  LConnTagsString=__new0  RConnTagsString=__new0  BranchType=R  Resistance=1e6  Inductance=1.6 / (120*pi) * 2  SetiL0=off  InitialCurrent=0  Capacitance=1e-6  Setx0=off  InitialVoltage=0  Measurements=None
      settings: SourceProductName=Simscape Electrical
  Sum : Sum  Inputs=|+-
  Voltage Measurement4 : powerlib/Measurements/Voltage Measurement  PhasorSimulation=off  OutputType=Complex  PSBequivalent=0
      settings: SourceProductName=Simscape Electrical
  Voltage Measurement5 : powerlib/Measurements/Voltage Measurement  PhasorSimulation=off  OutputType=Complex  PSBequivalent=0
      settings: SourceProductName=Simscape Electrical
  Voltage Measurement6 : powerlib/Measurements/Voltage Measurement  PhasorSimulation=off  OutputType=Complex  PSBequivalent=0
      settings: SourceProductName=Simscape Electrical
  " A" : PMIOPort  Tag=PMCPort  Side=Left
  " B" : PMIOPort  Tag=PMCPort  Port=2  Side=Left
  " C" : PMIOPort  Tag=PMCPort  Port=3  Side=Left
  wires:
  Magnitude-Angle to Complex1/1 -> Embedded MATLAB Function1/1(Vmeas)
  Memory3/1 -> Demux1/1, Fourier2/1
  "    4"/1 -> Magnitude-Angle to Complex1/1
  "    2"/1 -> Sum/1
  Voltage Measurement6/1 -> [vC]
  Demux1/1 -> Controlled Current Source/1
  [vC] -> Mux/3
  Sum/1 -> Memory4/1
  "    1"/1 -> Magnitude-Angle to Complex1/2
  Clock/1 -> Embedded MATLAB Function1/2(clock)
  Voltage Measurement5/1 -> [vB]
  Fourier1/2 -> "    2"/1
  Demux1/3 -> Controlled Current Source2/1
  Voltage Measurement4/1 -> [vA]
  Mux/1 -> Fourier/1
  Fourier/1 -> "    4"/1
  Demux1/2 -> Controlled Current Source1/1
  Fourier2/2 -> "    3"/1
  [del] -> Embedded MATLAB Function1/3(Ddel)
  Embedded MATLAB Function1/1(Iinjinst) -> Fourier1/1, Memory3/1
  [vA] -> Mux/1
  "    3"/1 -> Sum/2
  [vB] -> Mux/2
  Memory4/1 -> [del]
  Fourier/2 -> "    1"/1
  connections:
  Voltage Measurement5/LConn1 -- Rc+jXc2/LConn1 -- Controlled Current Source1/LConn1 -- " B"/RConn1 -- Rc+jXc1/RConn1 -- Controlled Current Source/RConn1 -- Voltage Measurement4/LConn2
  Voltage Measurement5/LConn2 -- Controlled Current Source1/RConn1 -- Rc+jXc2/RConn1 -- Controlled Current Source2/LConn1 -- " C"/RConn1 -- Voltage Measurement6/LConn1 -- Rc+jXc3/LConn1
  Voltage Measurement4/LConn1 -- Rc+jXc3/RConn1 -- Voltage Measurement6/LConn2 -- Controlled Current Source2/RConn1 -- Controlled Current Source/LConn1 -- " A"/RConn1 -- Rc+jXc1/LConn1

== system IEEE34bus_v2019b_Discrete_ZIPload/848 Y PQ ==
  "    1" : Gain  Gain=pi/180
  "    2" : Gain  Gain=pi/180
  "    3" : Gain  Gain=pi/180
  "    4" : Gain  Gain=1/sqrt(2)
  Clock : Clock
  Controlled Current Source : powerlib/Electrical Sources/Controlled Current Source  Initialize=off  Source_Type=AC  Amplitude=0  Phase=0  Frequency=0  Measurements=None
      settings: SourceProductName=Simscape Electrical
  Embedded MATLAB Function : MATLAB Function  TreatAsAtomicUnit=on
  Fourier : powerlib_meascontrol/Measurements/Fourier  Freq=60  n=1  InInit=[Vnom*sqrt(2) 0]  Ts=Ts
      settings: SourceProductName=Simscape Electrical
  Fourier1 : powerlib_meascontrol/Measurements/Fourier  Freq=60  n=1  InInit=[Vnom*sqrt(2) 0]  Ts=Ts
      settings: SourceProductName=Simscape Electrical
  Fourier2 : powerlib_meascontrol/Measurements/Fourier  Freq=60  n=1  InInit=[Vnom*sqrt(2) 0]  Ts=Ts
      settings: SourceProductName=Simscape Electrical
  Magnitude-Angle to Complex : MagnitudeAngleToComplex
  Memory1 : Memory
  Memory2 : Memory
  Rc+jXc1 : powerlib/Elements/Series RLC Branch  LConnTagsString=__new0  RConnTagsString=__new0  BranchType=R  Resistance=1e6  Inductance=1.6 / (120*pi) * 2  SetiL0=off  InitialCurrent=0  Capacitance=1e-6  Setx0=off  InitialVoltage=0  Measurements=None
      settings: SourceProductName=Simscape Electrical
  Sum : Sum  Inputs=|+-
  Voltage Measurement1 : powerlib/Measurements/Voltage Measurement  PhasorSimulation=off  OutputType=Complex  PSBequivalent=0
      settings: SourceProductName=Simscape Electrical
  " " : PMIOPort  Tag=PMCPort  Side=Left
  " 1" : PMIOPort  Tag=PMCPort  Port=2  Side=Right
  wires:
  Fourier1/2 -> "    1"/1
  Memory2/1 -> [del]
  Voltage Measurement1/1 -> [v]
  [v] -> Fourier/1
  "    1"/1 -> Sum/1
  Sum/1 -> Memory2/1
  Fourier/2 -> "    3"/1
  Fourier/1 -> "    4"/1
  [del] -> Embedded MATLAB Function/3(Ddel)
  Fourier2/2 -> "    2"/1
  Memory1/1 -> Controlled Current Source/1, Fourier2/1
  Embedded MATLAB Function/1(Iinjinst) -> Memory1/1, Fourier1/1
  Clock/1 -> Embedded MATLAB Function/2(clock)
  Magnitude-Angle to Complex/1 -> Embedded MATLAB Function/1(Vmeas)
  "    2"/1 -> Sum/2
  "    3"/1 -> Magnitude-Angle to Complex/2
  "    4"/1 -> Magnitude-Angle to Complex/1
  connections:
  " "/RConn1 -- Voltage Measurement1/LConn1 -- Controlled Current Source/LConn1 -- Rc+jXc1/LConn1
  Controlled Current Source/RConn1 -- Rc+jXc1/RConn1 -- Voltage Measurement1/LConn2 -- " 1"/RConn1
